simulink model "c4Sin_01_trans_002SampleTime"  (R2018b)
settings: Solver=VariableStepAuto  StartTime=0.0  StopTime=3.5  RelTol=1e-3  EnableMultiTasking=on
StopFcn:
  | c4erg=[tout,yout]
  | clear tout yout
settings Model: Creator=The MathWorks, Inc.  LastModifiedBy=Reichl
settings DataIOCC: LimitDataPoints=on  SaveFormat=Array
settings OptimizationCC: ExpressionDepthLimit=2147483647  LifeSpan=inf
settings DebuggingCC: UnderspecifiedInitializationDetection=Classic  MergeDetectMultiDrivingBlocksExec=none  InheritedTsInSrcMsg=none  FcnCallInpInsideContextMsg=warning  StateNameClashWarn=warning  SFUnexpectedBacktrackingDiag=warning  SFNoUnconditionalDefaultTransitionDiag=warning  SFExecutionAtInitializationDiag=none
settings HardwareCC: ProdBitPerPointer=32  ProdBitPerSizeT=32  ProdBitPerPtrDiffT=32  ProdLargestAtomicFloat=None  ProdIntDivRoundTo=Undefined  ProdEndianess=Unspecified  ProdWordSize=32  ProdHWDeviceType=32-bit Generic
settings ModelReferenceCC: PropagateSignalLabelsOutOfModel=off
settings SFSimCC: SimUseLocalCustomCode=off
settings RTWCC: RTWUseLocalCustomCode=off
settings CodeAppCC: StateflowObjectComments=on
settings GRTTargetCC: TargetLangStandard=C89/C90 (ANSI)  GeneratePreprocessorConditionals=Disable all  CombineOutputUpdateFcns=off  GRTInterface=on
settings ConfigComp: CovMetricSettings=dw  CovHtmlReporting=on  CovSaveCumulativeToWorkspaceVar=on  CovSaveSingleToWorkspaceVar=on  CovExternalEMLEnable=off

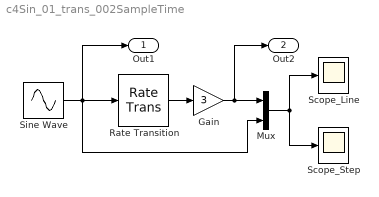
== system c4Sin_01_trans_002SampleTime ==
  Gain : Gain  Gain=3
  Mux : Mux  Inputs=2
  Rate Transition : RateTransition  OutPortSampleTime=0.02
  Scope_Line : Scope
  Scope_Step : Scope
  Sine Wave : Sin  SampleTime=0.1
  Out1 : Outport
  Out2 : Outport  Port=2
  wires:
  Sine Wave/1 -> Mux/2, Out1/1, Rate Transition/1
  Rate Transition/1 -> Gain/1
  Gain/1 -> Out2/1, Mux/1
  Mux/1 -> Scope_Line/1, Scope_Step/1
